simulink library "winch_ul"  (R2018b)
settings: Solver=VariableStepAuto  StartTime=0.0  StopTime=10.0  RelTol=1e-3
libraries: firstOrderFilter_ul x1
settings Model: Creator=mcobb  LastModifiedBy=mcobb

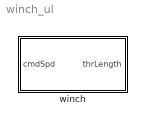
== system winch_ul ==
  winch : Subsystem  mask{initLength=0, maxSpd=1, tau=0, maxAccl=1}
      mask prompts: initLength "Initial tether length"; maxSpd "Max speed [m/s]"; tau "Time constant"; maxAccl "Max acceleration [m/s^2]"

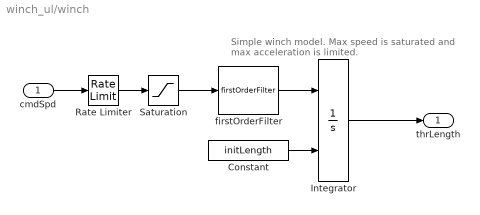
== system winch_ul/winch ==
  note: Simple winch model.  Max speed is saturated
      | and max acceleration is limited.
  cmdSpd : Inport  PortDimensions=1
  Constant : Constant  Value=initLength
  Integrator : Integrator  InitialConditionSource=external
  Rate Limiter : RateLimiter  RisingSlewLimit=maxAccl  FallingSlewLimit=-maxAccl  SampleTimeMode=inherited
  Saturation : Saturate  UpperLimit=maxSpd  LowerLimit=-maxSpd
  firstOrderFilter : firstOrderFilter_ul/firstOrderFilter  tau=tau  ic=0
  thrLength : Outport  PortDimensions=1
  wires:
  cmdSpd/1 -> Rate Limiter/1
  Integrator/1 -> thrLength/1
  Constant/1 -> Integrator/2
  Rate Limiter/1 -> Saturation/1
  Saturation/1 -> firstOrderFilter/1
  firstOrderFilter/1 -> Integrator/1
